simulink model "Reator_CSTR"  (R2021a)
settings: Solver=VariableStepAuto  StartTime=0.0  StopTime=tsim  RelTol=1e-3
values from neighbouring files (symbols this model uses):
  caf = 10    [mainCSTR.m]    (also in mainCSTR_control.m; mainControlCSTR.m; simulation_04_04_2024.mat)
  deltaE = 11843    [mainCSTR.m]    (also in mainCSTR_control.m; mainControlCSTR.m; simulation_04_04_2024.mat)
  deltaH = 5960    [mainCSTR.m]    (also in mainCSTR_control.m; mainControlCSTR.m; simulation_04_04_2024.mat)
  k0 = 9703*3600    (= 34930800)    [mainCSTR.m]    (also in mainCSTR_control.m; mainControlCSTR.m; simulation_04_04_2024.mat)
  R = 1.987    [mainCSTR.m]    (also in mainCSTR_control.m; mainControlCSTR.m; rga.m = pinv(G.').*G; simulation_04_04_2024.mat)
  rhocp = 500    [mainCSTR.m]    (also in mainCSTR_control.m; mainControlCSTR.m; simulation_04_04_2024.mat)
  Tf = 298    [mainCSTR.m]    (also in mainCSTR_control.m; mainControlCSTR.m; simulation_04_04_2024.mat)
  UAoV = 150    [mainCSTR.m]    (also in mainCSTR_control.m; mainControlCSTR.m; simulation_04_04_2024.mat)
  x0model = [5, 350]    [mainCSTR.m]    (also in mainCSTR_control.m = [8.5636  311.1710]; mainControlCSTR.m = [8.5636  311.1706]; simulation_04_04_2024.mat = [5 350])
settings Model: Creator=Aula  LastModifiedBy=Aula
settings DataIOCC: ReturnWorkspaceOutputs=off

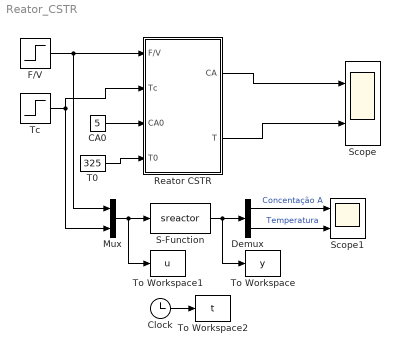
== system Reator_CSTR ==
  CA0 : Constant  Value=5
  Clock : Clock
  Demux : Demux  Outputs=2
  F/V : Step  Time=0  SampleTime=0
  Mux : Mux  Inputs=2
  Reator CSTR : Subsystem
  S-Function : S-Function  FunctionName=sreactor  Parameters=x0model,k0,deltaE,R,caf,Tf,deltaH,rhocp,UAoV  SFunctionDeploymentMode=off  EnableBusSupport=off
  Scope : Scope  NumInputPorts=2
  Scope1 : Scope  NumInputPorts=2
  T0 : Constant  Value=325
  Tc : Step  Time=0  After=298  SampleTime=0
  To Workspace : ToWorkspace  VariableName=y  SampleTime=-1
  "To Workspace1 " : ToWorkspace  VariableName=u  SampleTime=-1
  "To Workspace2 " : ToWorkspace  VariableName=t  SampleTime=-1
  wires:
  F/V/1 -> Mux/1, Reator CSTR/1(F/V)
  Tc/1 -> Reator CSTR/2(Tc), Mux/2
  Reator CSTR/1(CA) -> Scope/1
  Reator CSTR/2(T) -> Scope/2
  CA0/1 -> Reator CSTR/3(CA0)
  T0/1 -> Reator CSTR/4(T0)
  Mux/1 -> "To Workspace1 "/1, S-Function/1
  S-Function/1 -> To Workspace/1, Demux/1
  Demux/1 -> Scope1/1  "Concentação A"
  Demux/2 -> Scope1/2  "Temperatura"
  Clock/1 -> "To Workspace2 "/1

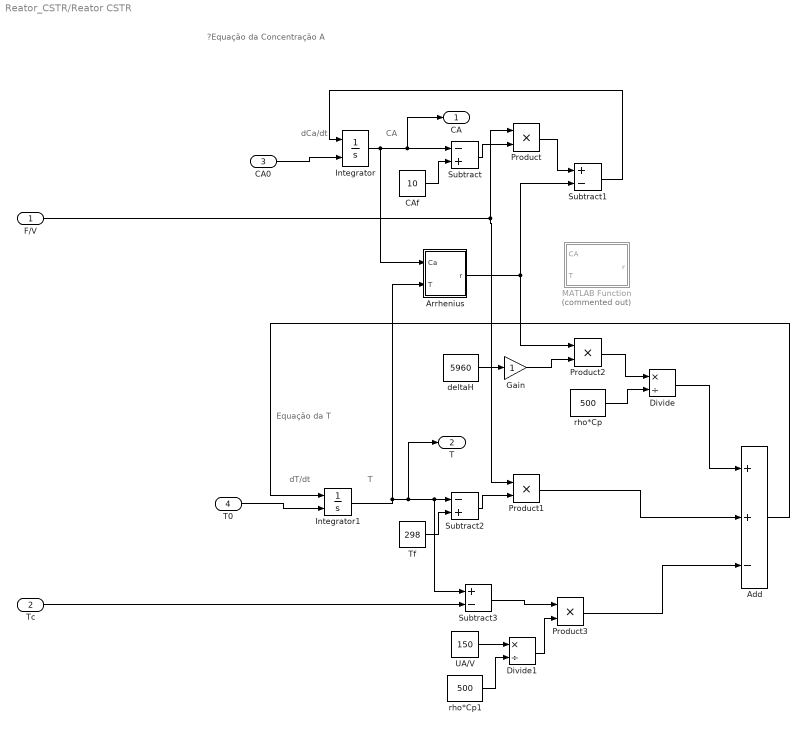
== system Reator_CSTR/Reator CSTR ==
  note: Equação da T
  note: ?Equação da Concentração A
  note: dT/dt
  note: T
  note: dCa/dt
  note: CA
  F/V : Inport
  Tc : Inport  Port=2
  CA0 : Inport  Port=3
  T0 : Inport  Port=4
  Add : Sum  Inputs=++-
  Arrhenius : Subsystem
  CAf : Constant  Value=10
  Divide : Product  Inputs=*/
  Divide1 : Product  Inputs=*/
  Gain : Gain
  Integrator : Integrator  InitialConditionSource=external  InitialCondition=5
  Integrator1 : Integrator  InitialConditionSource=external  InitialCondition=350
  MATLAB Function : MATLAB Function  Commented=on  TreatAsAtomicUnit=on
  Product{,1..3} (4 alike) : Product
  Subtract : Sum  Inputs=-+
  Subtract1 : Sum  Inputs=+-
  Subtract2 : Sum  Inputs=-+
  Subtract3 : Sum  Inputs=+-
  Tf : Constant  Value=298
  UA/V : Constant  Value=150
  deltaH : Constant  Value=5960
  rho*Cp : Constant  Value=500
  rho*Cp1 : Constant  Value=500
  CA : Outport
  T : Outport  Port=2
  wires:
  deltaH/1 -> Gain/1
  Tf/1 -> Subtract2/2
  rho*Cp/1 -> Divide/2
  UA/V/1 -> Divide1/1
  Integrator1/1 -> Arrhenius/2(T), T/1, Subtract3/1, Subtract2/1
  Divide1/1 -> Product3/2
  Integrator/1 -> Arrhenius/1(Ca), CA/1, Subtract/1
  rho*Cp1/1 -> Divide1/2
  Product/1 -> Subtract1/1
  Arrhenius/1(r) -> Product2/1, Subtract1/2
  F/V/1 -> Product1/1, Product/1
  Subtract3/1 -> Product3/1
  Subtract2/1 -> Product1/2
  CAf/1 -> Subtract/2
  Product2/1 -> Divide/1
  Subtract/1 -> Product/2
  Subtract1/1 -> Integrator/1
  Gain/1 -> Product2/2
  Divide/1 -> Add/1
  Add/1 -> Integrator1/1
  Product1/1 -> Add/2
  Product3/1 -> Add/3
  Tc/1 -> Subtract3/2
  CA0/1 -> Integrator/2
  T0/1 -> Integrator1/2

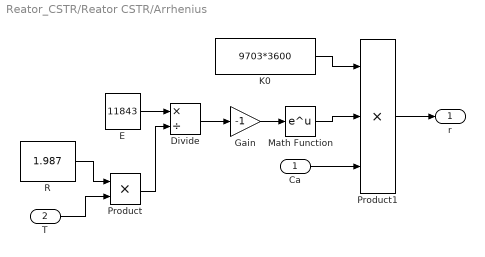
== system Reator_CSTR/Reator CSTR/Arrhenius ==
  Ca : Inport
  T : Inport  Port=2
  Divide : Product  Inputs=*/
  E : Constant  Value=11843
  Gain : Gain  Gain=-1
  K0 : Constant  Value=9703*3600
  Math Function : Math  SaturateOnIntegerOverflow=on
  Product : Product
  Product1 : Product  Inputs=3
  R : Constant  Value=1.987
  r : Outport
  wires:
  E/1 -> Divide/1
  Ca/1 -> Product1/3
  Gain/1 -> Math Function/1
  R/1 -> Product/1
  Product1/1 -> r/1
  Math Function/1 -> Product1/2
  K0/1 -> Product1/1
  T/1 -> Product/2
  Product/1 -> Divide/2
  Divide/1 -> Gain/1

== matlab function Reator_CSTR/Reator CSTR/MATLAB Function ==
  data: CA input; r output; T input
function r = Arrhenius(CA, T)
deltaE = 11.843;
R = 1.987*1000;
k0 = 9703 * 3600;

r = k0 * exp(-deltaE/(R*T))*CA;
